simulink model "exp4_p3A"  (R2018a)
settings: Solver=VariableStepAuto  StartTime=0.0  StopTime=10.0  RelTol=1e-3
libraries: powerlib x3
settings Model: Creator=Administrator  LastModifiedBy=Administrator

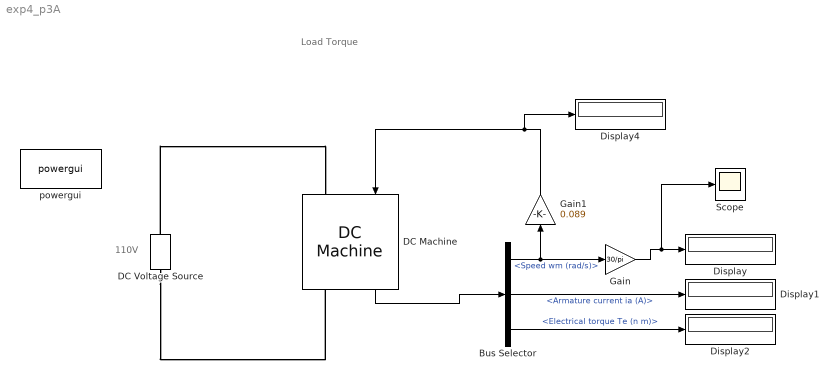
== system exp4_p3A ==
  note: 110V
  note: Load Torque
  Bus Selector : BusSelector  OutputSignals=Speed wm (rad/s),Armature current ia (A),Electrical torque Te (n m)
  DC Machine : powerlib/Machines/DC Machine  PresetModel=No  MechanicalLoad=Torque TL  FieldType=Permanent magnet  ShowDetailedParameters=on  MeasurementBus=off  RLa="[ 2  1.1e-3]"  RLf="[ 240  120]"  Laf=1.8  MachineConstant=Torque constant (N.m/A)  Ke=1.8  Kt=1.26  J=0.5  Bm=0  Tf=0  w0=1  Ifinit=1  TsPowergui=0  TsBlock=-1
  DC Voltage Source : powerlib/Electrical Sources/DC Voltage Source  Amplitude=110  Measurements=None
  Display{,1..2,4} (4 alike) : Display
  Gain : Gain  Gain=30/pi
  Gain1 : Gain  Gain=0.089
  Scope : Scope
  powergui : powerlib/powergui  Priority=1  SimulationMode=Continuous  SampleTime=50e-6  frequency=60  Iterations=50  frequencyindice=0  Pbase=100e6  ErrMax=1e-4  UnitsV=kV  UnitsW=MW  buscounter=0  FunctionMessages=off  echomessages=off  EnableUseOfTLC=off  CurrentSourceSwitches=off  DisableSnubberDevices=off  DisableRonSwitches=off  DisableVfSwitches=off  DisplayEquations=off  SolverType=Tustin/Backward Euler (TBE)  Interpol=off  ExternalGateDelay=off  methode=off  Ts=100  x0status=zero  SPID=on  SwTol=0  HookPort=off  RestoreLinks=warning  ResistiveCurrentMeasurement=off  Frange=[0:2:500]  Ylog=off  Xlog=on  ShowGrid=off  save=off  variable=ZData  structure=0  ZoomFFT=off  StartTime=0.0  cycles=1  DisplayStyle=1  fundamental=60  FreqAxis=off  MaxFrequency=1000  frequencyindicesteady=1  RmsSteady=1  display=off
  wires:
  Bus Selector/2 -> Display1/1  "<Armature current ia (A)>"
  Bus Selector/3 -> Display2/1  "<Electrical torque Te (n m)>"
  DC Machine/1 -> Bus Selector/1
  Gain/1 -> Scope/1, Display/1
  Bus Selector/1 -> Gain1/1, Gain/1  "<Speed wm (rad/s)>"
  Gain1/1 -> Display4/1, DC Machine/1
  connections:
  DC Voltage Source/RConn1 -- DC Machine/LConn1
  DC Voltage Source/LConn1 -- DC Machine/RConn1
